simulink model "C28069_LLC_ePWM_V8_230307_PhaeShiftWorking"  (R2022b)
settings: Solver=FixedStepAuto  StartTime=0.0  StopTime=10  RelTol=1e-3  EnableMultiTasking=on
model workspace (MAT data in the model file):
  Comp_DAC = 512
undefined symbols (not defined in the file or in its folder): Down, GPTRIP1SEL, GPTRIP2SEL, PWM_Control, PWM_Gen, PWM_Gen1, SCI_A_Transmit, SCI_A_Transmit_Current_Suffix, SCI_A_Transmit_Duty_Suffix, SCI_A_Transmit_Freq_Suffix, SCI_A_Transmit_OVPFlag_Suffix, SCI_A_Transmit_PFC_Suffix, SCI_A_Transmit_SS_Suffix, SCI_A_Transmit_TBPHS_Suffix, SCI_A_Transmit_VADC_Suffix, SCI_A_Transmit_VAvg_Suffix, SCI_A_Transmit_VBAT_Suffix, SCI_A_Transmit_VBATRef_Suffix, SCI_A_Transmit_Vo_Suffix, TZ1, TZ2, u1, Up
libraries: c2802xlib x92, c280xlib x39, simulink x36, c2000lib x1
(part 10 of 18)

== system C28069_LLC_ePWM_V8_230307_PhaeShiftWorking/CloseLoop & Update @ ADCINT, 50kHz/Control/Frequency Update/Simulink Function3 ==
  note: Added Trigger
  note: Fixing deadtime to 250ns
  note: Control CMPA/B to Zero
      | When the input is <1KHz
      | (To switch off ePWM)
  note: Frequency Input Selection
  note: Original
  PWM_Control : TriggerPort  TriggerType=function-call  IsSimulinkFunction=on  FunctionName=PWM_Control  FunctionVisibility=scoped  VariantControl=(inherit)
  CMPA : Display
  CMPA1 : Display
  CMPB : Display
  CMPB1 : Display
  Constant : Constant  Value=100
  Constant1 : Constant
  Constant2 : Constant  Value=0
  Constant3 : Constant  Value=50
  Constant4 : Constant
  Dead time (%) : Display
  Dead time (sec) : Constant  Value=250E-9
  Divide : Product  Inputs=*/
  Gain1 : Gain  Gain=1000
  Gain2 : Gain  Gain=100
  Product1 : Product  Inputs=3
  Product2 : Product
  Product3 : Product
  Product4 : Product
  Subsystem1 : Subsystem
  Subtract : Sum  Inputs=+-
  Switch : Switch  Criteria=u2 > Threshold  Threshold=1  SaturateOnIntegerOverflow=off  InputSameDT=off
  Switch1 : Switch  Criteria=u2 > Threshold  OutDataTypeStr=double  SaturateOnIntegerOverflow=off  InputSameDT=off
  TBPRD : Display
  ePWM1 : c2802xlib/ePWM  PwmType=C2000  useModule=ePWM6  ePWMxLINKTBPRD=Not Linked  periodUnits=Clock cycles  timerSource=Input port  timerPeriod_clk=294  timerPeriod_sec=0.0001  tbshadow=Counter equals to zero  countingMode=Up-Down  phaseActiveEnable=Disable  phaseDirection=Count down after sync  phaseActive=0  synchronizationEnable=off  dcaevt1Sync=off  dcbevt1Sync=off  synchronizationOption=Disable  dcbevt1SyncOut=off  dcaevt1SyncOut=off  cmpdSyncOut=off  cmpcSyncOut=off  cmpbSyncOut=off  zeroSyncOut=off  swfSyncOut=off  perSynchronizationOption=Counter equals to period (CTR=PRD)  clockPrescale=1  HSclockPrescale=1  enswap=off  ePWMxAStatus=on  ePWMxAactionLogic1=Do nothing  ePWMxAactionLogic2=Do nothing  ePWMxAactionLogic3=Set  ePWMxAactionLogic4=Do nothing  ePWMxAactionLogic5=Clear  ePWMxAactionLogic6=Do nothing  ePWMxACSFenable=off  ePWMxACSFvalue=Forcing disable  ePWMxASFreload=Zero  ePWMxBStatus=on  ePWMxBactionLogic1=Do nothing  ePWMxBactionLogic2=Do nothing  ePWMxBactionLogic3=Do nothing  ePWMxBactionLogic4=Clear  ePWMxBactionLogic5=Do nothing  ePWMxBactionLogic6=Set  ePWMxBCSFenable=off  ePWMxBCSFvalue=Forcing disable  ePWMxBSFreload=Zero  ePWNxBOutWay=off  ePWMxLINKCMPA=Not Linked  CMPAUnits=Clock cycles  CMPASource=Input port  CMPAValue_per=50  CMPAValue_clk=0  enCMPAshadow=Counter equals to zero (CTR=Zero)  ePWMxLINKCMPB=Not Linked  CMPBUnits=Clock cycles  CMPBSource=Input port  CMPBValue_per=50  CMPBValue_clk=0  enCMPBshadow=Counter equals to zero (CTR=Zero)  ePWMxLINKCMPC=Not Linked  CMPCUnits=Clock cycles  CMPCSource=Specify via dialog  CMPCValue_per=50  CMPCValue_clk=32000  enCMPCshadow=Counter equals to zero (CTR=Zero)  ePWMxLINKCMPD=Not Linked  CMPDUnits=Clock cycles  CMPDSource=Specify via dialog  CMPDValue_per=50  CMPDValue_clk=32000  enCMPDshadow=Counter equals to zero (CTR=Zero)  enableDBePWMxA=off  enableDBePWMxB=off  enhalfcycle=off  DBpolarity=Active high complementary (AHC)  DBedgeDelay=Positive  DBSource_ePWMxA=ePWMxA  DBSource_ePWMxB=ePWMxA  DBPeriodUnits=Clock cycles  DBperiodSource=Input port  REDperiod=10  FEDperiod=10  REDperiod_sec=0  FEDperiod_sec=0  LoadModeDBRED=Immediate without using shadow  LoadModeDBFED=Immediate without using shadow  adcstartModuleA=off  adcrequestEventA=First event  adcstartEventA=Counter equals to zero (CTR=Zero)  adcstartEventA_type2=Digital Compare Module A Event 1 start of conversion (DCAEVT1.soc)  adcstartModuleB=off  adcrequestEventB=First event  adcstartEventB=Counter equals to zero (CTR=Zero)  adcstartEventB_type2=Counter equals to zero (CTR=Zero)  intEn=off  intPrd=First event  intSel=Counter equals to zero (CTR=Zero)  intSel_type2=Counter equals to zero (CTR=Zero)  hrpe=off  enHRPWM=off  HRPWM_LoadMode=Counter equals to period (CTR=PRD)  HRPWM_CTLMode=Duty or Period control mode  HRPWM_EDGMode=Both edge  hrpeb=off  enHRPWMB=off  HRPWM_LoadModeB=Counter equals to zero (CTR=ZERO)  HRPWM_CTLModeB=Duty or Period control mode  HRPWM_EDGModeB=Both edge  enHRDBRED=off  enHRDBFED=off  enSFO=on  enautoconv=on  chopperEnable=off  chopperFrequency=1  chopperFirstwidth=1  chopperDuty=12.5%  tripZonesource=Specify via dialog  tzselOSHT1=off  tzselOSHT2=off  tzselOSHT3=off  tzselOSHDCAEV1=off  tzselOSHDCBEV1=off  tzselCBC1=off  tzselCBC2=off  tzselCBC3=off  tzselCBCDCAEV2=off  tzselCBCDCBEV2=off  tzselOSHT4=off  tzselOSHT5=off  tzselOSHT6=off  tzselCBC4=off  tzselCBC5=off  tzselCBC6=off  enTzOstIntr=off  enTzCbcIntr=off  enTzDCAEVT1Intr=off  enTzDCAEVT2Intr=off  enTzDCBEVT1Intr=off  enTzDCBEVT2Intr=off  ePWMxAforced=No action  ePWMxBforced=No action  DCAEVT1forced=Low  DCBEVT1forced=Low  DCAEVT2forced=No action  DCBEVT2forced=No action  dcah=COMP1OUT input  dcal=Trip Zone 1 input (TZ1)  dcbh=COMP1OUT input  dcbl=Trip Zone 1 input (TZ1)  dcah_type2=GPTRIP1SEL/(TZ1)  dcal_type2=GPTRIP2SEL/(TZ2)  dcbh_type2=GPTRIP1SEL/(TZ1)  dcbl_type2=GPTRIP2SEL/(TZ2)  gendcaevt1=DCAH=high and DCAL=don't care  gendcaevt2=Event disabled  gendcbevt1=DCBH=high and DCBL=don't care  gendcbevt2=Event disabled  dcaevt1src=DCAEVT1 with sync  dcaevt2src=DCAEVT2 with sync  dcbevt1src=DCBEVT1 with sync  dcbevt2src=DCBEVT2 with sync  pulsesel=Counter equals to zero (CTR=Zero)  blankinv=off  blankoffset=0  blankwidth=0  evsrcsel=Filtered version of DCAEVT1 (DCAEVT1FILT)  encape=off
      settings: LibrarySourceBlock=c2806xlib/ePWM
  ePWM4 : c2802xlib/ePWM  PwmType=C2000  useModule=ePWM5  ePWMxLINKTBPRD=Not Linked  periodUnits=Clock cycles  timerSource=Input port  timerPeriod_clk=294  timerPeriod_sec=0.0001  tbshadow=Counter equals to zero  countingMode=Up-Down  phaseActiveEnable=Disable  phaseDirection=Count down after sync  phaseActive=0  synchronizationEnable=off  dcaevt1Sync=off  dcbevt1Sync=off  synchronizationOption=Disable  dcbevt1SyncOut=off  dcaevt1SyncOut=off  cmpdSyncOut=off  cmpcSyncOut=off  cmpbSyncOut=off  zeroSyncOut=off  swfSyncOut=off  perSynchronizationOption=Counter equals to period (CTR=PRD)  clockPrescale=1  HSclockPrescale=1  enswap=off  ePWMxAStatus=on  ePWMxAactionLogic1=Do nothing  ePWMxAactionLogic2=Do nothing  ePWMxAactionLogic3=Set  ePWMxAactionLogic4=Do nothing  ePWMxAactionLogic5=Clear  ePWMxAactionLogic6=Do nothing  ePWMxACSFenable=off  ePWMxACSFvalue=Forcing disable  ePWMxASFreload=Zero  ePWMxBStatus=on  ePWMxBactionLogic1=Do nothing  ePWMxBactionLogic2=Do nothing  ePWMxBactionLogic3=Do nothing  ePWMxBactionLogic4=Clear  ePWMxBactionLogic5=Do nothing  ePWMxBactionLogic6=Set  ePWMxBCSFenable=off  ePWMxBCSFvalue=Forcing disable  ePWMxBSFreload=Zero  ePWNxBOutWay=off  ePWMxLINKCMPA=Not Linked  CMPAUnits=Clock cycles  CMPASource=Input port  CMPAValue_per=50  CMPAValue_clk=0  enCMPAshadow=Counter equals to zero (CTR=Zero)  ePWMxLINKCMPB=Not Linked  CMPBUnits=Clock cycles  CMPBSource=Input port  CMPBValue_per=50  CMPBValue_clk=0  enCMPBshadow=Counter equals to zero (CTR=Zero)  ePWMxLINKCMPC=Not Linked  CMPCUnits=Clock cycles  CMPCSource=Specify via dialog  CMPCValue_per=50  CMPCValue_clk=32000  enCMPCshadow=Counter equals to zero (CTR=Zero)  ePWMxLINKCMPD=Not Linked  CMPDUnits=Clock cycles  CMPDSource=Specify via dialog  CMPDValue_per=50  CMPDValue_clk=32000  enCMPDshadow=Counter equals to zero (CTR=Zero)  enableDBePWMxA=off  enableDBePWMxB=off  enhalfcycle=off  DBpolarity=Active high complementary (AHC)  DBedgeDelay=Positive  DBSource_ePWMxA=ePWMxA  DBSource_ePWMxB=ePWMxA  DBPeriodUnits=Clock cycles  DBperiodSource=Input port  REDperiod=10  FEDperiod=10  REDperiod_sec=0  FEDperiod_sec=0  LoadModeDBRED=Immediate without using shadow  LoadModeDBFED=Immediate without using shadow  adcstartModuleA=on  adcrequestEventA=First event  adcstartEventA=Counter equals to zero (CTR=Zero)  adcstartEventA_type2=Digital Compare Module A Event 1 start of conversion (DCAEVT1.soc)  adcstartModuleB=off  adcrequestEventB=First event  adcstartEventB=Counter equals to zero (CTR=Zero)  adcstartEventB_type2=Counter equals to zero (CTR=Zero)  intEn=on  intPrd=First event  intSel=Counter equals to zero (CTR=Zero)  intSel_type2=Counter equals to zero (CTR=Zero)  hrpe=off  enHRPWM=off  HRPWM_LoadMode=Counter equals to period (CTR=PRD)  HRPWM_CTLMode=Duty or Period control mode  HRPWM_EDGMode=Both edge  hrpeb=off  enHRPWMB=off  HRPWM_LoadModeB=Counter equals to zero (CTR=ZERO)  HRPWM_CTLModeB=Duty or Period control mode  HRPWM_EDGModeB=Both edge  enHRDBRED=off  enHRDBFED=off  enSFO=on  enautoconv=on  chopperEnable=off  chopperFrequency=1  chopperFirstwidth=1  chopperDuty=12.5%  tripZonesource=Specify via dialog  tzselOSHT1=off  tzselOSHT2=off  tzselOSHT3=off  tzselOSHDCAEV1=off  tzselOSHDCBEV1=off  tzselCBC1=off  tzselCBC2=off  tzselCBC3=off  tzselCBCDCAEV2=off  tzselCBCDCBEV2=off  tzselOSHT4=off  tzselOSHT5=off  tzselOSHT6=off  tzselCBC4=off  tzselCBC5=off  tzselCBC6=off  enTzOstIntr=off  enTzCbcIntr=off  enTzDCAEVT1Intr=off  enTzDCAEVT2Intr=off  enTzDCBEVT1Intr=off  enTzDCBEVT2Intr=off  ePWMxAforced=No action  ePWMxBforced=No action  DCAEVT1forced=Low  DCBEVT1forced=Low  DCAEVT2forced=No action  DCBEVT2forced=No action  dcah=COMP1OUT input  dcal=Trip Zone 1 input (TZ1)  dcbh=COMP1OUT input  dcbl=Trip Zone 1 input (TZ1)  dcah_type2=GPTRIP1SEL/(TZ1)  dcal_type2=GPTRIP2SEL/(TZ2)  dcbh_type2=GPTRIP1SEL/(TZ1)  dcbl_type2=GPTRIP2SEL/(TZ2)  gendcaevt1=DCAH=high and DCAL=don't care  gendcaevt2=Event disabled  gendcbevt1=DCBH=high and DCBL=don't care  gendcbevt2=Event disabled  dcaevt1src=DCAEVT1 with sync  dcaevt2src=DCAEVT2 with sync  dcbevt1src=DCBEVT1 with sync  dcbevt2src=DCBEVT2 with sync  pulsesel=Counter equals to zero (CTR=Zero)  blankinv=off  blankoffset=0  blankwidth=0  evsrcsel=Filtered version of DCAEVT1 (DCAEVT1FILT)  encape=off
      settings: LibrarySourceBlock=c2806xlib/ePWM
  original : c2802xlib/ePWM  Commented=on  PwmType=C2000  useModule=ePWM6  ePWMxLINKTBPRD=Not Linked  periodUnits=Clock cycles  timerSource=Input port  timerPeriod_clk=294  timerPeriod_sec=0.0001  tbshadow=Counter equals to zero  countingMode=Up-Down  phaseActiveEnable=Disable  phaseDirection=Count down after sync  phaseActive=0  synchronizationEnable=off  dcaevt1Sync=off  dcbevt1Sync=off  synchronizationOption=Disable  dcbevt1SyncOut=off  dcaevt1SyncOut=off  cmpdSyncOut=off  cmpcSyncOut=off  cmpbSyncOut=off  zeroSyncOut=off  swfSyncOut=off  perSynchronizationOption=Counter equals to period (CTR=PRD)  clockPrescale=1  HSclockPrescale=1  enswap=off  ePWMxAStatus=on  ePWMxAactionLogic1=Do nothing  ePWMxAactionLogic2=Do nothing  ePWMxAactionLogic3=Set  ePWMxAactionLogic4=Do nothing  ePWMxAactionLogic5=Clear  ePWMxAactionLogic6=Do nothing  ePWMxACSFenable=off  ePWMxACSFvalue=Forcing disable  ePWMxASFreload=Zero  ePWMxBStatus=on  ePWMxBactionLogic1=Do nothing  ePWMxBactionLogic2=Do nothing  ePWMxBactionLogic3=Do nothing  ePWMxBactionLogic4=Clear  ePWMxBactionLogic5=Do nothing  ePWMxBactionLogic6=Set  ePWMxBCSFenable=off  ePWMxBCSFvalue=Forcing disable  ePWMxBSFreload=Zero  ePWNxBOutWay=off  ePWMxLINKCMPA=Not Linked  CMPAUnits=Clock cycles  CMPASource=Input port  CMPAValue_per=50  CMPAValue_clk=12  enCMPAshadow=Counter equals to zero (CTR=Zero)  ePWMxLINKCMPB=Not Linked  CMPBUnits=Clock cycles  CMPBSource=Input port  CMPBValue_per=50  CMPBValue_clk=283  enCMPBshadow=Counter equals to zero (CTR=Zero)  ePWMxLINKCMPC=Not Linked  CMPCUnits=Clock cycles  CMPCSource=Specify via dialog  CMPCValue_per=50  CMPCValue_clk=32000  enCMPCshadow=Counter equals to zero (CTR=Zero)  ePWMxLINKCMPD=Not Linked  CMPDUnits=Clock cycles  CMPDSource=Specify via dialog  CMPDValue_per=50  CMPDValue_clk=32000  enCMPDshadow=Counter equals to zero (CTR=Zero)  enableDBePWMxA=off  enableDBePWMxB=off  enhalfcycle=off  DBpolarity=Active high complementary (AHC)  DBedgeDelay=Positive  DBSource_ePWMxA=ePWMxA  DBSource_ePWMxB=ePWMxA  DBPeriodUnits=Clock cycles  DBperiodSource=Input port  REDperiod=10  FEDperiod=10  REDperiod_sec=0  FEDperiod_sec=0  LoadModeDBRED=Immediate without using shadow  LoadModeDBFED=Immediate without using shadow  adcstartModuleA=off  adcrequestEventA=First event  adcstartEventA=Counter equals to zero (CTR=Zero)  adcstartEventA_type2=Digital Compare Module A Event 1 start of conversion (DCAEVT1.soc)  adcstartModuleB=off  adcrequestEventB=First event  adcstartEventB=Counter equals to zero (CTR=Zero)  adcstartEventB_type2=Counter equals to zero (CTR=Zero)  intEn=off  intPrd=First event  intSel=Counter equals to zero (CTR=Zero)  intSel_type2=Counter equals to zero (CTR=Zero)  hrpe=off  enHRPWM=off  HRPWM_LoadMode=Counter equals to period (CTR=PRD)  HRPWM_CTLMode=Duty or Period control mode  HRPWM_EDGMode=Both edge  hrpeb=off  enHRPWMB=off  HRPWM_LoadModeB=Counter equals to zero (CTR=ZERO)  HRPWM_CTLModeB=Duty or Period control mode  HRPWM_EDGModeB=Both edge  enHRDBRED=off  enHRDBFED=off  enSFO=on  enautoconv=on  chopperEnable=off  chopperFrequency=1  chopperFirstwidth=1  chopperDuty=12.5%  tripZonesource=Specify via dialog  tzselOSHT1=off  tzselOSHT2=off  tzselOSHT3=off  tzselOSHDCAEV1=off  tzselOSHDCBEV1=off  tzselCBC1=off  tzselCBC2=off  tzselCBC3=off  tzselCBCDCAEV2=off  tzselCBCDCBEV2=off  tzselOSHT4=off  tzselOSHT5=off  tzselOSHT6=off  tzselCBC4=off  tzselCBC5=off  tzselCBC6=off  enTzOstIntr=off  enTzCbcIntr=off  enTzDCAEVT1Intr=off  enTzDCAEVT2Intr=off  enTzDCBEVT1Intr=off  enTzDCBEVT2Intr=off  ePWMxAforced=No action  ePWMxBforced=No action  DCAEVT1forced=Low  DCBEVT1forced=Low  DCAEVT2forced=No action  DCBEVT2forced=No action  dcah=COMP1OUT input  dcal=Trip Zone 1 input (TZ1)  dcbh=COMP1OUT input  dcbl=Trip Zone 1 input (TZ1)  dcah_type2=GPTRIP1SEL/(TZ1)  dcal_type2=GPTRIP2SEL/(TZ2)  dcbh_type2=GPTRIP1SEL/(TZ1)  dcbl_type2=GPTRIP2SEL/(TZ2)  gendcaevt1=DCAH=high and DCAL=don't care  gendcaevt2=Event disabled  gendcbevt1=DCBH=high and DCBL=don't care  gendcbevt2=Event disabled  dcaevt1src=DCAEVT1 with sync  dcaevt2src=DCAEVT2 with sync  dcbevt1src=DCBEVT1 with sync  dcbevt2src=DCBEVT2 with sync  pulsesel=Counter equals to zero (CTR=Zero)  blankinv=off  blankoffset=0  blankwidth=0  evsrcsel=Filtered version of DCAEVT1 (DCAEVT1FILT)  encape=off
      settings: LibrarySourceBlock=c2806xlib/ePWM
  u : ArgIn  DisableCoverage=on  ArgumentName=u
  u1 : ArgIn  DisableCoverage=on  Port=2  OutDataTypeStr=uint16  ArgumentName=u1
  wires:
  Switch1/1 -> Subsystem1/1(Frequency(kHz)), Switch/2, Gain1/1
  u/1 -> Switch1/1, Switch1/2
  Constant3/1 -> Subsystem1/2(Duty(%))
  Divide/1 -> Product2/2
  Product2/1 -> Subtract/2, Product3/1, CMPA/1
  Constant/1 -> Divide/2
  Subtract/1 -> Product4/1, CMPB/1
  Subsystem1/1(Out1) -> Product2/1, Subtract/1, ePWM4/1, ePWM1/1, TBPRD/1
  Gain1/1 -> Product1/1
  Dead time (sec)/1 -> Product1/2
  Constant1/1 -> Switch/1
  Constant2/1 -> Switch/3
  Switch/1 -> Product3/2, Product4/2
  Product3/1 -> ePWM1/2, ePWM4/2, CMPA1/1
  Product4/1 -> CMPB1/1, ePWM4/3, ePWM1/3
  Constant4/1 -> Switch1/3
  u1/1 -> Product1/3
  Product1/1 -> Gain2/1
  Gain2/1 -> Dead time (%)/1, Divide/1

== system C28069_LLC_ePWM_V8_230307_PhaeShiftWorking/CloseLoop & Update @ ADCINT, 50kHz/Control/Get AVG2/MovingAverage_7Window ==
  note: Average the value
  In1 : Inport
  Delay12 : Delay  DelayLength=5
  Delay13 : Delay  DelayLength=6
  Delay14 : Delay  DelayLength=1
  Delay15 : Delay
  Delay16 : Delay  DelayLength=3
  Delay17 : Delay  DelayLength=4
  Gain2 : Gain  Gain=1/7  OutDataTypeStr=uint16
  Sum2 : Sum  Inputs=|+++++++
  Out1 : Outport
  wires:
  Delay17/1 -> Sum2/5
  Gain2/1 -> Out1/1, Delay13/1, Delay12/1, Delay17/1, Delay16/1, Delay15/1, Delay14/1
  In1/1 -> Sum2/1
  Delay12/1 -> Sum2/6
  Delay13/1 -> Sum2/7
  Delay16/1 -> Sum2/4
  Delay15/1 -> Sum2/3
  Delay14/1 -> Sum2/2
  Sum2/1 -> Gain2/1

== system C28069_LLC_ePWM_V8_230307_PhaeShiftWorking/CloseLoop & Update @ ADCINT, 50kHz/Frequency Update/Simulink Function1/Subsystem1 ==
  Frequency(kHz) : Inport  OutDataTypeStr=double
  Duty(%) : Inport  Port=2
  Constant1 : Constant  Value=90E6
  Divide : Product  Inputs=*/  RndMeth=Zero  SaturateOnIntegerOverflow=on
  Gain : Gain  Gain=1000
  Gain1 : Gain  Gain=1/100
  Gain2 : Gain  Gain=0.5
  Product : Product
  Product1 : Product
  Up-Down Counter : Constant  Value=2
  Out1 : Outport
  Out2 : Outport  Port=2
  Out3 : Outport  Port=3
  wires:
  Gain2/1 -> Out3/1
  Gain1/1 -> Product1/2
  Product1/1 -> Gain2/1, Out2/1
  Duty(%)/1 -> Gain1/1
  Divide/1 -> Out1/1, Product1/1
  Constant1/1 -> Divide/1
  Frequency(kHz)/1 -> Gain/1
  Product/1 -> Divide/2
  Gain/1 -> Product/1
  Up-Down Counter/1 -> Product/2

== system C28069_LLC_ePWM_V8_230307_PhaeShiftWorking/CloseLoop & Update @ ADCINT, 50kHz/Frequency Update/Simulink Function2/Subsystem1 ==
  Frequency(kHz) : Inport  OutDataTypeStr=double
  Duty(%) : Inport  Port=2
  Constant1 : Constant  Value=90E6
  Divide : Product  Inputs=*/  RndMeth=Zero  SaturateOnIntegerOverflow=on
  Gain : Gain  Gain=1000
  Gain1 : Gain  Gain=1/100
  Gain2 : Gain  Gain=0.5
  Product : Product
  Product1 : Product
  Up-Down Counter : Constant  Value=2
  Out1 : Outport
  Out2 : Outport  Port=2
  Out3 : Outport  Port=3
  wires:
  Up-Down Counter/1 -> Product/2
  Gain/1 -> Product/1
  Product/1 -> Divide/2
  Frequency(kHz)/1 -> Gain/1
  Constant1/1 -> Divide/1
  Divide/1 -> Product1/1, Out1/1
  Duty(%)/1 -> Gain1/1
  Product1/1 -> Out2/1, Gain2/1
  Gain1/1 -> Product1/2
  Gain2/1 -> Out3/1

== system C28069_LLC_ePWM_V8_230307_PhaeShiftWorking/CloseLoop & Update @ ADCINT, 50kHz/Frequency Update1/Simulink Function1/Subsystem1 ==
  Frequency(kHz) : Inport  OutDataTypeStr=double
  Duty(%) : Inport  Port=2
  Constant1 : Constant  Value=90E6
  Divide : Product  Inputs=*/  RndMeth=Zero  SaturateOnIntegerOverflow=on
  Gain : Gain  Gain=1000
  Gain1 : Gain  Gain=1/100
  Gain2 : Gain  Gain=0.5
  Product : Product
  Product1 : Product
  Up-Down Counter : Constant  Value=2
  Out1 : Outport
  Out2 : Outport  Port=2
  Out3 : Outport  Port=3
  wires:
  Up-Down Counter/1 -> Product/2
  Gain/1 -> Product/1
  Product/1 -> Divide/2
  Frequency(kHz)/1 -> Gain/1
  Constant1/1 -> Divide/1
  Divide/1 -> Product1/1, Out1/1
  Duty(%)/1 -> Gain1/1
  Product1/1 -> Out2/1, Gain2/1
  Gain1/1 -> Product1/2
  Gain2/1 -> Out3/1

== system C28069_LLC_ePWM_V8_230307_PhaeShiftWorking/CloseLoop & Update @ ADCINT, 50kHz/Frequency Update1/Simulink Function2/Subsystem1 ==
  Frequency(kHz) : Inport
  Duty(%) : Inport  Port=2
  Constant1 : Constant  Value=90E6
  Divide : Product  Inputs=*/  RndMeth=Zero  SaturateOnIntegerOverflow=on
  Gain : Gain  Gain=1000
  Gain1 : Gain  Gain=1/100
  Gain2 : Gain  Gain=0.5
  Product : Product
  Product1 : Product
  Up-Down Counter : Constant  Value=2
  Out1 : Outport
  Out2 : Outport  Port=2
  Out3 : Outport  Port=3
  wires:
  Up-Down Counter/1 -> Product/2
  Gain/1 -> Product/1
  Product/1 -> Divide/2
  Frequency(kHz)/1 -> Gain/1
  Constant1/1 -> Divide/1
  Divide/1 -> Product1/1, Out1/1
  Duty(%)/1 -> Gain1/1
  Product1/1 -> Out2/1, Gain2/1
  Gain1/1 -> Product1/2
  Gain2/1 -> Out3/1

== system C28069_LLC_ePWM_V8_230307_PhaeShiftWorking/CloseLoop & Update @ ADCINT, 50kHz/Frequency Update1/Simulink Function3/Subsystem1 ==
  Frequency(kHz) : Inport  OutDataTypeStr=double
  Duty(%) : Inport  Port=2
  Constant1 : Constant  Value=90E6
  Divide : Product  Inputs=*/  RndMeth=Zero  SaturateOnIntegerOverflow=on
  Gain : Gain  Gain=1000
  Gain1 : Gain  Gain=1/100
  Gain2 : Gain  Gain=0.5
  Product : Product
  Product1 : Product
  Up-Down Counter : Constant  Value=2
  Out1 : Outport
  Out2 : Outport  Port=2
  Out3 : Outport  Port=3
  wires:
  Up-Down Counter/1 -> Product/2
  Gain/1 -> Product/1
  Product/1 -> Divide/2
  Frequency(kHz)/1 -> Gain/1
  Constant1/1 -> Divide/1
  Divide/1 -> Product1/1, Out1/1
  Duty(%)/1 -> Gain1/1
  Product1/1 -> Out2/1, Gain2/1
  Gain1/1 -> Product1/2
  Gain2/1 -> Out3/1

== system C28069_LLC_ePWM_V8_230307_PhaeShiftWorking/GetADC Measurement @50KHz3/Frequency Update/Simulink Function1/Subsystem1 ==
  Frequency(kHz) : Inport  OutDataTypeStr=double
  Duty(%) : Inport  Port=2
  Constant1 : Constant  Value=90E6
  Divide : Product  Inputs=*/  RndMeth=Zero  SaturateOnIntegerOverflow=on
  Gain : Gain  Gain=1000
  Gain1 : Gain  Gain=1/100
  Gain2 : Gain  Gain=0.5
  Product : Product
  Product1 : Product
  Up-Down Counter : Constant  Value=2
  Out1 : Outport
  Out2 : Outport  Port=2
  Out3 : Outport  Port=3
  wires:
  Gain2/1 -> Out3/1
  Gain1/1 -> Product1/2
  Product1/1 -> Gain2/1, Out2/1
  Duty(%)/1 -> Gain1/1
  Divide/1 -> Out1/1, Product1/1
  Constant1/1 -> Divide/1
  Frequency(kHz)/1 -> Gain/1
  Product/1 -> Divide/2
  Gain/1 -> Product/1
  Up-Down Counter/1 -> Product/2

== system C28069_LLC_ePWM_V8_230307_PhaeShiftWorking/GetADC Measurement @50KHz3/Frequency Update/Simulink Function2/Subsystem1 ==
  Frequency(kHz) : Inport
  Duty(%) : Inport  Port=2
  Constant1 : Constant  Value=90E6
  Divide : Product  Inputs=*/  RndMeth=Zero  SaturateOnIntegerOverflow=on
  Gain : Gain  Gain=1000
  Gain1 : Gain  Gain=1/100
  Gain2 : Gain  Gain=0.5
  Product : Product
  Product1 : Product
  Up-Down Counter : Constant  Value=2
  Out1 : Outport
  Out2 : Outport  Port=2
  Out3 : Outport  Port=3
  wires:
  Gain2/1 -> Out3/1
  Gain1/1 -> Product1/2
  Product1/1 -> Gain2/1, Out2/1
  Duty(%)/1 -> Gain1/1
  Divide/1 -> Out1/1, Product1/1
  Constant1/1 -> Divide/1
  Frequency(kHz)/1 -> Gain/1
  Product/1 -> Divide/2
  Gain/1 -> Product/1
  Up-Down Counter/1 -> Product/2

== system C28069_LLC_ePWM_V8_230307_PhaeShiftWorking/GetADC Measurement @50KHz3/Frequency Update/Simulink Function3/Subsystem1 ==
  Frequency(kHz) : Inport  OutDataTypeStr=double
  Duty(%) : Inport  Port=2
  Constant1 : Constant  Value=90E6
  Divide : Product  Inputs=*/  RndMeth=Zero  SaturateOnIntegerOverflow=on
  Gain : Gain  Gain=1000
  Gain1 : Gain  Gain=1/100
  Gain2 : Gain  Gain=0.5
  Product : Product
  Product1 : Product
  Up-Down Counter : Constant  Value=2
  Out1 : Outport
  Out2 : Outport  Port=2
  Out3 : Outport  Port=3
  wires:
  Gain2/1 -> Out3/1
  Gain1/1 -> Product1/2
  Product1/1 -> Gain2/1, Out2/1
  Duty(%)/1 -> Gain1/1
  Divide/1 -> Out1/1, Product1/1
  Constant1/1 -> Divide/1
  Frequency(kHz)/1 -> Gain/1
  Product/1 -> Divide/2
  Gain/1 -> Product/1
  Up-Down Counter/1 -> Product/2

== system C28069_LLC_ePWM_V8_230307_PhaeShiftWorking/GetADC, FaultProtection, SoftStart  @5KHz/Fault Protection @ 5KHz/If Action Subsystem/OCP ==
  note: 1900 = @>1.9A Load will trigger
  note: False
  note: Average the value
  note: True
  function : TriggerPort  TriggerType=function-call  VariantControl=(inherit)
  ADC : c2802xlib/ADC  Commented=on  blkParamProc=C2000  ADCModule=1  samplingMode=Single sample mode  ADCResolution=12-bit (Single-ended input)  useSOC1=SOC0  useSOC2=SOC0_SOC1  SOCAcquisitionWindow=7  SOCTriggerSource=ePWM5_ADCSOCA  SOCInterruptTrigger=No ADCINT  Ts=-1  dType=uint16  postInterrupt=off  interruptSel=ADCINT1  ADCINTContinuous=off  endma=off  chdma=1  conv1=ADCINA2  conv2=ADCINA0 and ADCINB0  conv1_Type4=ADCIN0  conv2_Type4=ADCIN0 and ADCIN1
      settings: LibrarySourceBlock=c2806xlib/ADC
  Constant3 : Constant  Value=0  OutDataTypeStr=single
  Data Store Read : DataStoreRead  DataStoreName=OCP_Flag  IndexOptions=Index vector (dialog)  Indices=1  OutputSizes=1
  Data Store Read1 : DataStoreRead  DataStoreName=IoutCurrentBAT_Value  IndexOptions=Index vector (dialog)  Indices=1  OutputSizes=1
  Data Store Write2 : DataStoreWrite  DataStoreName=OCP_Flag  IndexOptions=Index vector (dialog)  Indices=1  OutputSizes=1
  Data Type Conversion1 : DataTypeConversion  OutDataTypeStr=double  SaturateOnIntegerOverflow=off  RndMeth=Floor
  Delay : Delay  Commented=on  DelayLength=1
  Delay1 : Delay  Commented=on
  Delay2 : Delay  Commented=on  DelayLength=3
  Delay3 : Delay  Commented=on  DelayLength=4
  Delay4 : Delay  Commented=on  DelayLength=5
  Display7 : Display
  Gain : Gain  Commented=on  Gain=1/6  OutDataTypeStr=uint16
  Sum : Sum  Commented=on  Inputs=|++++++
  Switch : Switch  Criteria=u2 > Threshold  Threshold=2100  OutDataTypeStr=single  SaturateOnIntegerOverflow=off  InputSameDT=off
  wires:
  Data Store Read1/1 -> Switch/2, Display7/1
  Delay4/1 -> Sum/6
  Delay3/1 -> Sum/5
  Gain/1 -> Delay/1, Delay1/1, Delay2/1, Delay3/1, Delay4/1
  Delay/1 -> Sum/2
  Delay1/1 -> Sum/3
  Delay2/1 -> Sum/4
  Sum/1 -> Gain/1
  Data Type Conversion1/1 -> Data Store Write2/1
  Data Store Read/1 -> Switch/3
  Constant3/1 -> Switch/1
  Switch/1 -> Data Type Conversion1/1
  ADC/1 -> Sum/1

== system C28069_LLC_ePWM_V8_230307_PhaeShiftWorking/GetADC, FaultProtection, SoftStart  @5KHz/Fault Protection @ 5KHz/If Action Subsystem/OVP ==
  note: True
  note: Average the value
  note: False
  note: >92Vdc will trigger
  function : TriggerPort  TriggerType=function-call  VariantControl=(inherit)
  ADC : c2802xlib/ADC  Commented=on  blkParamProc=C2000  ADCModule=1  samplingMode=Single sample mode  ADCResolution=12-bit (Single-ended input)  useSOC1=SOC0  useSOC2=SOC0_SOC1  SOCAcquisitionWindow=7  SOCTriggerSource=ePWM5_ADCSOCA  SOCInterruptTrigger=No ADCINT  Ts=-1  dType=uint16  postInterrupt=off  interruptSel=ADCINT1  ADCINTContinuous=off  endma=off  chdma=1  conv1=ADCINA2  conv2=ADCINA0 and ADCINB0  conv1_Type4=ADCIN0  conv2_Type4=ADCIN0 and ADCIN1
      settings: LibrarySourceBlock=c2806xlib/ADC
  Constant3 : Constant  Value=0  OutDataTypeStr=single
  Data Store Read : DataStoreRead  DataStoreName=OVP_Flag  IndexOptions=Index vector (dialog)  Indices=1  OutputSizes=1
  Data Store Read1 : DataStoreRead  DataStoreName=VBAT_Value  IndexOptions=Index vector (dialog)  Indices=1  OutputSizes=1
  Data Store Write2 : DataStoreWrite  DataStoreName=OVP_Flag  IndexOptions=Index vector (dialog)  Indices=1  OutputSizes=1
  Data Type Conversion1 : DataTypeConversion  OutDataTypeStr=double  SaturateOnIntegerOverflow=off  RndMeth=Floor
  Delay : Delay  Commented=on  DelayLength=1
  Delay1 : Delay  Commented=on
  Delay2 : Delay  Commented=on  DelayLength=3
  Delay3 : Delay  Commented=on  DelayLength=4
  Delay4 : Delay  Commented=on  DelayLength=5
  Display7 : Display
  Gain : Gain  Commented=on  Gain=1/6  OutDataTypeStr=uint16
  Sum : Sum  Commented=on  Inputs=|++++++
  Switch : Switch  Criteria=u2 > Threshold  Threshold=35  OutDataTypeStr=single  SaturateOnIntegerOverflow=off  InputSameDT=off
  wires:
  ADC/1 -> Sum/1
  Switch/1 -> Data Type Conversion1/1
  Constant3/1 -> Switch/1
  Data Store Read/1 -> Switch/3
  Data Type Conversion1/1 -> Data Store Write2/1
  Sum/1 -> Gain/1
  Delay2/1 -> Sum/4
  Delay1/1 -> Sum/3
  Delay/1 -> Sum/2
  Gain/1 -> Delay4/1, Delay3/1, Delay2/1, Delay1/1, Delay/1
  Delay3/1 -> Sum/5
  Delay4/1 -> Sum/6
  Data Store Read1/1 -> Display7/1, Switch/2

== system C28069_LLC_ePWM_V8_230307_PhaeShiftWorking/GetADC, FaultProtection, SoftStart  @5KHz/Fault Protection @ 5KHz/If Action Subsystem/TestToCheckOVPFlag ==
  note: Comment out GPIO14 when flash to MB, as SCI_B using GPIO14
  note: Test to check if this OVP_Flag is working
  function : TriggerPort  TriggerType=function-call  VariantControl=(inherit)
  Data Store Read : DataStoreRead  DataStoreName=OVP_Flag  IndexOptions=Index vector (dialog)  Indices=1  OutputSizes=1
  GPIO14 Test : c280xlib/Digital Output  GPIO_Number=GPIO8~GPIO15  GPIO_Bit0=off  GPIO_BIT0_Toggle=off  GPIO_Bit1=off  GPIO_BIT1_Toggle=off  GPIO_Bit2=off  GPIO_BIT2_Toggle=off  GPIO_Bit3=off  GPIO_BIT3_Toggle=off  GPIO_Bit4=off  GPIO_BIT4_Toggle=off  GPIO_Bit5=off  GPIO_BIT5_Toggle=off  GPIO_Bit6=on  GPIO_BIT6_Toggle=off  GPIO_Bit7=off  GPIO_BIT7_Toggle=off
  wires:
  Data Store Read/1 -> GPIO14 Test/1

== system C28069_LLC_ePWM_V8_230307_PhaeShiftWorking/GetADC, FaultProtection, SoftStart  @5KHz/Fault Protection @ 5KHz1/If Action Subsystem/OCP ==
  note: 1900 = @>1.9A Load will trigger
  note: False
  note: Average the value
  note: True
  function : TriggerPort  TriggerType=function-call  VariantControl=(inherit)
  ADC : c2802xlib/ADC  Commented=on  blkParamProc=C2000  ADCModule=1  samplingMode=Single sample mode  ADCResolution=12-bit (Single-ended input)  useSOC1=SOC0  useSOC2=SOC0_SOC1  SOCAcquisitionWindow=7  SOCTriggerSource=ePWM5_ADCSOCA  SOCInterruptTrigger=No ADCINT  Ts=-1  dType=uint16  postInterrupt=off  interruptSel=ADCINT1  ADCINTContinuous=off  endma=off  chdma=1  conv1=ADCINA2  conv2=ADCINA0 and ADCINB0  conv1_Type4=ADCIN0  conv2_Type4=ADCIN0 and ADCIN1
      settings: LibrarySourceBlock=c2806xlib/ADC
  Constant3 : Constant  Value=0  OutDataTypeStr=single
  Data Store Read : DataStoreRead  DataStoreName=OCP_Flag  IndexOptions=Index vector (dialog)  Indices=1  OutputSizes=1
  Data Store Read1 : DataStoreRead  DataStoreName=IoutCurrentBAT_Value  IndexOptions=Index vector (dialog)  Indices=1  OutputSizes=1
  Data Store Write2 : DataStoreWrite  DataStoreName=OCP_Flag  IndexOptions=Index vector (dialog)  Indices=1  OutputSizes=1
  Data Type Conversion1 : DataTypeConversion  OutDataTypeStr=double  SaturateOnIntegerOverflow=off  RndMeth=Floor
  Delay : Delay  Commented=on  DelayLength=1
  Delay1 : Delay  Commented=on
  Delay2 : Delay  Commented=on  DelayLength=3
  Delay3 : Delay  Commented=on  DelayLength=4
  Delay4 : Delay  Commented=on  DelayLength=5
  Display7 : Display
  Gain : Gain  Commented=on  Gain=1/6  OutDataTypeStr=uint16
  Sum : Sum  Commented=on  Inputs=|++++++
  Switch : Switch  Criteria=u2 > Threshold  Threshold=2100  OutDataTypeStr=single  SaturateOnIntegerOverflow=off  InputSameDT=off
  wires:
  Data Store Read1/1 -> Switch/2, Display7/1
  Delay4/1 -> Sum/6
  Delay3/1 -> Sum/5
  Gain/1 -> Delay/1, Delay1/1, Delay2/1, Delay3/1, Delay4/1
  Delay/1 -> Sum/2
  Delay1/1 -> Sum/3
  Delay2/1 -> Sum/4
  Sum/1 -> Gain/1
  Data Type Conversion1/1 -> Data Store Write2/1
  Data Store Read/1 -> Switch/3
  Constant3/1 -> Switch/1
  Switch/1 -> Data Type Conversion1/1
  ADC/1 -> Sum/1

== system C28069_LLC_ePWM_V8_230307_PhaeShiftWorking/GetADC, FaultProtection, SoftStart  @5KHz/Fault Protection @ 5KHz1/If Action Subsystem/OVP ==
  note: True
  note: Average the value
  note: False
  note: >92Vdc will trigger
  function : TriggerPort  TriggerType=function-call  VariantControl=(inherit)
  ADC : c2802xlib/ADC  Commented=on  blkParamProc=C2000  ADCModule=1  samplingMode=Single sample mode  ADCResolution=12-bit (Single-ended input)  useSOC1=SOC0  useSOC2=SOC0_SOC1  SOCAcquisitionWindow=7  SOCTriggerSource=ePWM5_ADCSOCA  SOCInterruptTrigger=No ADCINT  Ts=-1  dType=uint16  postInterrupt=off  interruptSel=ADCINT1  ADCINTContinuous=off  endma=off  chdma=1  conv1=ADCINA2  conv2=ADCINA0 and ADCINB0  conv1_Type4=ADCIN0  conv2_Type4=ADCIN0 and ADCIN1
      settings: LibrarySourceBlock=c2806xlib/ADC
  Constant3 : Constant  Value=0  OutDataTypeStr=single
  Data Store Read : DataStoreRead  DataStoreName=OVP_Flag  IndexOptions=Index vector (dialog)  Indices=1  OutputSizes=1
  Data Store Read1 : DataStoreRead  DataStoreName=VBAT_Value  IndexOptions=Index vector (dialog)  Indices=1  OutputSizes=1
  Data Store Write2 : DataStoreWrite  DataStoreName=OVP_Flag  IndexOptions=Index vector (dialog)  Indices=1  OutputSizes=1
  Data Type Conversion1 : DataTypeConversion  OutDataTypeStr=double  SaturateOnIntegerOverflow=off  RndMeth=Floor
  Delay : Delay  Commented=on  DelayLength=1
  Delay1 : Delay  Commented=on
  Delay2 : Delay  Commented=on  DelayLength=3
  Delay3 : Delay  Commented=on  DelayLength=4
  Delay4 : Delay  Commented=on  DelayLength=5
  Display7 : Display
  Gain : Gain  Commented=on  Gain=1/6  OutDataTypeStr=uint16
  Sum : Sum  Commented=on  Inputs=|++++++
  Switch : Switch  Criteria=u2 > Threshold  Threshold=35  OutDataTypeStr=single  SaturateOnIntegerOverflow=off  InputSameDT=off
  wires:
  ADC/1 -> Sum/1
  Switch/1 -> Data Type Conversion1/1
  Constant3/1 -> Switch/1
  Data Store Read/1 -> Switch/3
  Data Type Conversion1/1 -> Data Store Write2/1
  Sum/1 -> Gain/1
  Delay2/1 -> Sum/4
  Delay1/1 -> Sum/3
  Delay/1 -> Sum/2
  Gain/1 -> Delay4/1, Delay3/1, Delay2/1, Delay1/1, Delay/1
  Delay3/1 -> Sum/5
  Delay4/1 -> Sum/6
  Data Store Read1/1 -> Display7/1, Switch/2

== system C28069_LLC_ePWM_V8_230307_PhaeShiftWorking/GetADC, FaultProtection, SoftStart  @5KHz/Fault Protection @ 5KHz1/If Action Subsystem/TestToCheckOVPFlag ==
  note: Comment out GPIO14 when flash to MB, as SCI_B using GPIO14
  note: Test to check if this OVP_Flag is working
  function : TriggerPort  TriggerType=function-call  VariantControl=(inherit)
  Data Store Read : DataStoreRead  DataStoreName=OVP_Flag  IndexOptions=Index vector (dialog)  Indices=1  OutputSizes=1
  GPIO14 Test : c280xlib/Digital Output  GPIO_Number=GPIO8~GPIO15  GPIO_Bit0=off  GPIO_BIT0_Toggle=off  GPIO_Bit1=off  GPIO_BIT1_Toggle=off  GPIO_Bit2=off  GPIO_BIT2_Toggle=off  GPIO_Bit3=off  GPIO_BIT3_Toggle=off  GPIO_Bit4=off  GPIO_BIT4_Toggle=off  GPIO_Bit5=off  GPIO_BIT5_Toggle=off  GPIO_Bit6=on  GPIO_BIT6_Toggle=off  GPIO_Bit7=off  GPIO_BIT7_Toggle=off
  wires:
  Data Store Read/1 -> GPIO14 Test/1

== system C28069_LLC_ePWM_V8_230307_PhaeShiftWorking/GetADC, FaultProtection, SoftStart  @5KHz/Frequency Update/Simulink Function1/Subsystem1 ==
  Frequency(kHz) : Inport  OutDataTypeStr=double
  Duty(%) : Inport  Port=2
  Constant1 : Constant  Value=90E6
  Divide : Product  Inputs=*/  RndMeth=Zero  SaturateOnIntegerOverflow=on
  Gain : Gain  Gain=1000
  Gain1 : Gain  Gain=1/100
  Gain2 : Gain  Gain=0.5
  Product : Product
  Product1 : Product
  Up-Down Counter : Constant  Value=2
  Out1 : Outport
  Out2 : Outport  Port=2
  Out3 : Outport  Port=3
  wires:
  Up-Down Counter/1 -> Product/2
  Gain/1 -> Product/1
  Product/1 -> Divide/2
  Frequency(kHz)/1 -> Gain/1
  Constant1/1 -> Divide/1
  Divide/1 -> Product1/1, Out1/1
  Duty(%)/1 -> Gain1/1
  Product1/1 -> Out2/1, Gain2/1
  Gain1/1 -> Product1/2
  Gain2/1 -> Out3/1

== system C28069_LLC_ePWM_V8_230307_PhaeShiftWorking/GetADC, FaultProtection, SoftStart  @5KHz/Frequency Update/Simulink Function2/Subsystem1 ==
  Frequency(kHz) : Inport
  Duty(%) : Inport  Port=2
  Constant1 : Constant  Value=90E6
  Divide : Product  Inputs=*/  RndMeth=Zero  SaturateOnIntegerOverflow=on
  Gain : Gain  Gain=1000
  Gain1 : Gain  Gain=1/100
  Gain2 : Gain  Gain=0.5
  Product : Product
  Product1 : Product
  Up-Down Counter : Constant  Value=2
  Out1 : Outport
  Out2 : Outport  Port=2
  Out3 : Outport  Port=3
  wires:
  Up-Down Counter/1 -> Product/2
  Gain/1 -> Product/1
  Product/1 -> Divide/2
  Frequency(kHz)/1 -> Gain/1
  Constant1/1 -> Divide/1
  Divide/1 -> Product1/1, Out1/1
  Duty(%)/1 -> Gain1/1
  Product1/1 -> Out2/1, Gain2/1
  Gain1/1 -> Product1/2
  Gain2/1 -> Out3/1

== system C28069_LLC_ePWM_V8_230307_PhaeShiftWorking/GetADC, FaultProtection, SoftStart  @5KHz/Frequency Update/Simulink Function3/Subsystem1 ==
  Frequency(kHz) : Inport  OutDataTypeStr=double
  Duty(%) : Inport  Port=2
  Constant1 : Constant  Value=90E6
  Divide : Product  Inputs=*/  RndMeth=Zero  SaturateOnIntegerOverflow=on
  Gain : Gain  Gain=1000
  Gain1 : Gain  Gain=1/100
  Gain2 : Gain  Gain=0.5
  Product : Product
  Product1 : Product
  Up-Down Counter : Constant  Value=2
  Out1 : Outport
  Out2 : Outport  Port=2
  Out3 : Outport  Port=3
  wires:
  Up-Down Counter/1 -> Product/2
  Gain/1 -> Product/1
  Product/1 -> Divide/2
  Frequency(kHz)/1 -> Gain/1
  Constant1/1 -> Divide/1
  Divide/1 -> Product1/1, Out1/1
  Duty(%)/1 -> Gain1/1
  Product1/1 -> Out2/1, Gain2/1
  Gain1/1 -> Product1/2
  Gain2/1 -> Out3/1

== system C28069_LLC_ePWM_V8_230307_PhaeShiftWorking/GetADC, FaultProtection, SoftStart  @5KHz/SoftStart/If Action Subsystem/ReservseSoftStart ==
  function : TriggerPort  TriggerType=function-call  VariantControl=(inherit)
  Chart1 : Stateflow chart  TreatAsAtomicUnit=on
  Constant : Constant  Value=160  OutDataTypeStr=double  SampleTime=Inf
  Constant1 : Constant  Value=200  OutDataTypeStr=double  SampleTime=Inf
  Constant2 : Constant  SampleTime=Inf
  Data Store Read : DataStoreRead  DataStoreName=PFC_OK  IndexOptions=Index vector (dialog)  Indices=1  OutputSizes=1
  Data Store Write1 : DataStoreWrite  DataStoreName=SoftStart_OK_Signal  IndexOptions=Index vector (dialog)  Indices=1  OutputSizes=1
  Data Store Write2 : DataStoreWrite  DataStoreName=Freq_Value  IndexOptions=Index vector (dialog)  Indices=1  OutputSizes=1
  Data Store Write3 : DataStoreWrite  DataStoreName=Duty_Value  IndexOptions=Index vector (dialog)  Indices=1  OutputSizes=1
  Data Type Conversion : DataTypeConversion  OutDataTypeStr=uint16  SaturateOnIntegerOverflow=off  RndMeth=Floor
  Data Type Conversion1 : DataTypeConversion  OutDataTypeStr=uint16  SaturateOnIntegerOverflow=off  RndMeth=Floor
  Data Type Conversion2 : DataTypeConversion  Commented=on  OutDataTypeStr=uint8  SaturateOnIntegerOverflow=off  RndMeth=Floor
  ms : Constant  Commented=on  Value=15  SampleTime=Inf
  wires:
  Constant1/1 -> Chart1/3(Resonant_Frequency)
  Constant/1 -> Chart1/2(Initial_Frequency)
  Data Type Conversion/1 -> Data Store Write2/1
  Chart1/3(Frequency_Adjusted) -> Data Type Conversion/1
  Chart1/1(SoftStart_OK) -> Data Store Write1/1
  Chart1/2(Duty_Adjusted) -> Data Type Conversion1/1
  Data Type Conversion1/1 -> Data Store Write3/1
  Data Store Read/1 -> Chart1/1(PFC_OK)

== system C28069_LLC_ePWM_V8_230307_PhaeShiftWorking/GetADC, FaultProtection, SoftStart  @5KHz/SoftStart/If Action Subsystem/SoftStart ==
  function : TriggerPort  TriggerType=function-call  VariantControl=(inherit)
  Chart1 : Stateflow chart  TreatAsAtomicUnit=on
  Constant : Constant  Value=153  OutDataTypeStr=double  SampleTime=Inf
  Constant1 : Constant  Value=130  OutDataTypeStr=double  SampleTime=Inf
  Data Store Read : DataStoreRead  DataStoreName=PFC_OK  IndexOptions=Index vector (dialog)  Indices=1  OutputSizes=1
  Data Store Write1 : DataStoreWrite  DataStoreName=SoftStart_OK_Signal  IndexOptions=Index vector (dialog)  Indices=1  OutputSizes=1
  Data Store Write2 : DataStoreWrite  DataStoreName=Freq_Value  IndexOptions=Index vector (dialog)  Indices=1  OutputSizes=1
  wires:
  Chart1/1(SoftStart_OK) -> Data Store Write1/1
  Chart1/2(Frequency_Adjusted) -> Data Store Write2/1
  Constant/1 -> Chart1/2(Initial_Frequency)
  Constant1/1 -> Chart1/3(Resonant_Frequency)
  Data Store Read/1 -> Chart1/1(PFC_OK)

== system C28069_LLC_ePWM_V8_230307_PhaeShiftWorking/GetADC, FaultProtection, SoftStart  @5KHz/SoftStart1/If Action Subsystem/ReservseSoftStart1 ==
  function : TriggerPort  TriggerType=function-call  VariantControl=(inherit)
  Chart1 : Stateflow chart  TreatAsAtomicUnit=on
  Constant : Constant  Value=160  OutDataTypeStr=double  SampleTime=Inf
  Constant1 : Constant  Value=200  OutDataTypeStr=double  SampleTime=Inf
  Constant2 : Constant  SampleTime=Inf
  Data Store Read : DataStoreRead  DataStoreName=PFC_OK  IndexOptions=Index vector (dialog)  Indices=1  OutputSizes=1
  Data Store Write1 : DataStoreWrite  DataStoreName=SoftStart_OK_Signal  IndexOptions=Index vector (dialog)  Indices=1  OutputSizes=1
  Data Store Write2 : DataStoreWrite  DataStoreName=Freq_Value  IndexOptions=Index vector (dialog)  Indices=1  OutputSizes=1
  Data Store Write3 : DataStoreWrite  DataStoreName=Duty_Value  IndexOptions=Index vector (dialog)  Indices=1  OutputSizes=1
  Data Type Conversion : DataTypeConversion  OutDataTypeStr=uint16  SaturateOnIntegerOverflow=off  RndMeth=Floor
  Data Type Conversion1 : DataTypeConversion  OutDataTypeStr=uint16  SaturateOnIntegerOverflow=off  RndMeth=Floor
  Data Type Conversion2 : DataTypeConversion  Commented=on  OutDataTypeStr=uint8  SaturateOnIntegerOverflow=off  RndMeth=Floor
  ms : Constant  Commented=on  Value=15  SampleTime=Inf
  wires:
  Constant1/1 -> Chart1/3(Resonant_Frequency)
  Constant/1 -> Chart1/2(Initial_Frequency)
  Data Type Conversion/1 -> Data Store Write2/1
  Chart1/3(Frequency_Adjusted) -> Data Type Conversion/1
  Chart1/1(SoftStart_OK) -> Data Store Write1/1
  Chart1/2(Duty_Adjusted) -> Data Type Conversion1/1
  Data Type Conversion1/1 -> Data Store Write3/1
  Data Store Read/1 -> Chart1/1(PFC_OK)

== system C28069_LLC_ePWM_V8_230307_PhaeShiftWorking/GetADC, FaultProtection, SoftStart  @5KHz/SoftStart1/If Action Subsystem/SoftStart1 ==
  function : TriggerPort  TriggerType=function-call  VariantControl=(inherit)
  Chart : Stateflow chart  TreatAsAtomicUnit=on
  Chart1 : Stateflow chart  Commented=on  TreatAsAtomicUnit=on
  Constant : Constant  Commented=on  Value=153  OutDataTypeStr=double  SampleTime=Inf
  Constant1 : Constant  Commented=on  Value=130  OutDataTypeStr=double  SampleTime=Inf
  Constant2 : Constant  Value=15  OutDataTypeStr=double  SampleTime=Inf
  Data Store Read : DataStoreRead  Commented=on  DataStoreName=PFC_OK  IndexOptions=Index vector (dialog)  Indices=1  OutputSizes=1
  Data Store Read1 : DataStoreRead  DataStoreName=PFC_OK  IndexOptions=Index vector (dialog)  Indices=1  OutputSizes=1
  Data Store Read2 : DataStoreRead  DataStoreName=VBAT_Value  IndexOptions=Index vector (dialog)  Indices=1  OutputSizes=1
  Data Store Write : DataStoreWrite  DataStoreName=VBAT_Ref_Value  IndexOptions=Index vector (dialog)  Indices=1  OutputSizes=1
  Data Store Write1 : DataStoreWrite  Commented=on  DataStoreName=SoftStart_OK_Signal  IndexOptions=Index vector (dialog)  Indices=1  OutputSizes=1
  Data Store Write2 : DataStoreWrite  Commented=on  DataStoreName=Freq_Value  IndexOptions=Index vector (dialog)  Indices=1  OutputSizes=1
  Data Store Write3 : DataStoreWrite  DataStoreName=SoftStart_OK_Signal  IndexOptions=Index vector (dialog)  Indices=1  OutputSizes=1
  GPIO21 : c280xlib/Digital Output  GPIO_Number=GPIO16~GPIO23  GPIO_Bit0=off  GPIO_BIT0_Toggle=off  GPIO_Bit1=off  GPIO_BIT1_Toggle=off  GPIO_Bit2=off  GPIO_BIT2_Toggle=off  GPIO_Bit3=off  GPIO_BIT3_Toggle=off  GPIO_Bit4=off  GPIO_BIT4_Toggle=off  GPIO_Bit5=on  GPIO_BIT5_Toggle=off  GPIO_Bit6=off  GPIO_BIT6_Toggle=off  GPIO_Bit7=off  GPIO_BIT7_Toggle=off
  wires:
  Chart1/1(SoftStart_OK) -> Data Store Write1/1
  Chart1/2(Frequency_Adjusted) -> Data Store Write2/1
  Constant/1 -> Chart1/2(Initial_Frequency)
  Constant1/1 -> Chart1/3(Resonant_Frequency)
  Data Store Read/1 -> Chart1/1(PFC_OK)
  Data Store Read1/1 -> GPIO21/1, Chart/1(PFC_OK)
  Constant2/1 -> Chart/3(VBAT_Ref)
  Data Store Read2/1 -> Chart/2(VBAT_Value)
  Chart/1(VBAT_Ref_adjusted) -> Data Store Write/1
  Chart/2(SoftStart_OK) -> Data Store Write3/1

== system C28069_LLC_ePWM_V8_230307_PhaeShiftWorking/GetADC, FaultProtection, SoftStart  @5KHz/UpdatePWM/Close Loop Regulation/If Action Subsystem ==
  note: Take note : All of them are ADC values.
  note: Voltage regulation for LLC (Not done yet)
  note: Regulation the Output Voltage and Sweeping the frequency accordingly to meet the output voltage.
      | Than if hit the 'max' frequency, it will trigger to reduce the duty cycle.
  Action Port : ActionPort  ActionPortLabel=if((u1 == 1) & (u2 == 1))
  Chart : Stateflow chart  TreatAsAtomicUnit=on
  Constant70 : Constant  Value=100  OutDataTypeStr=double
  Constant71 : Constant  Value=180  OutDataTypeStr=double
  Data Store Read : DataStoreRead  DataStoreName=VBAT_Value  IndexOptions=Index vector (dialog)  Indices=1  OutputSizes=1
  Data Store Read1 : DataStoreRead  DataStoreName=Freq_Value  IndexOptions=Index vector (dialog)  Indices=1  OutputSizes=1
  Data Store Write1 : DataStoreWrite  DataStoreName=Freq_Value  IndexOptions=Index vector (dialog)  Indices=1  OutputSizes=1
  Data Type Conversion : DataTypeConversion  OutDataTypeStr=double  SaturateOnIntegerOverflow=off  RndMeth=Floor
  Saturation Dynamic1 : simulink/Discontinuities/Saturation Dynamic  OutMin=[]  OutMax=[]  OutDataTypeStr=double  OutputDataTypeScalingMode=single  OutDataType=single  OutScaling=2^-10  DoSatur=off
  Testing30Vout ReferencePoint : Constant  Value=25  OutDataTypeStr=double
  V_err : Sum  Inputs=|+-  AccumDataTypeStr=double  OutDataTypeStr=double
  wires:
  Constant71/1 -> [Max_Freq]
  Testing30Vout ReferencePoint/1 -> V_err/1
  Data Store Read/1 -> Data Type Conversion/1
  Saturation Dynamic1/1 -> Data Store Write1/1
  V_err/1 -> Chart/1(input_u)
  [Max_Freq] -> Saturation Dynamic1/1
  [Min_Freq] -> Saturation Dynamic1/3
  Chart/1(output_y) -> Saturation Dynamic1/2
  Constant70/1 -> [Min_Freq]
  Data Store Read1/1 -> Chart/2(prev_freq)
  Data Type Conversion/1 -> V_err/2
